simulink model "test"  (R2019a)
settings: Solver=VariableStepAuto  StartTime=0.0  StopTime=inf  RelTol=1e-3
settings Model: EnablePacing=on  Creator=wuyuanyi  LastModifiedBy=wuyuanyi

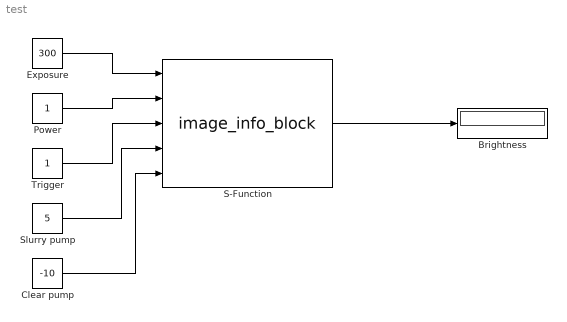
== system test ==
  Brightness : Display
  Clear pump : Constant  Value=-10
  Exposure : Constant  Value=300
  Power : Constant
  S-Function : S-Function  FunctionName=image_info_block  Parameters=1,int32(5),int32(1)  SFunctionDeploymentMode=off  EnableBusSupport=off
  Slurry pump : Constant  Value=5
  Trigger : Constant
  wires:
  S-Function/1 -> Brightness/1
  Exposure/1 -> S-Function/1
  Power/1 -> S-Function/2
  Trigger/1 -> S-Function/3
  Slurry pump/1 -> S-Function/4
  Clear pump/1 -> S-Function/5
